simulink model "Model_14Bus_Microgrid_R2018"  (R2018b)
settings: Solver=ode23tb  StartTime=0.0  StopTime=0.35  MaxStep=1e-2  RelTol=1e-3
InitFcn:
  | Set_parameters_R2018
StopFcn:
  | Save_Data;
  | Graphics;
values from neighbouring files (symbols this model uses):
  Clink = Ceq*2    (= 0.217013888889)    [Set_parameters_R2017b.m]    (also in Set_parameters_R2018.m)
  dis1 = 0.15    [Set_parameters_R2017b.m]    (also in Set_parameters_R2018.m)
  dis10 = 6    [Set_parameters_R2017b.m]    (also in Set_parameters_R2018.m)
  dis11 = 3    [Set_parameters_R2017b.m]    (also in Set_parameters_R2018.m)
  dis12 = 6    [Set_parameters_R2017b.m]    (also in Set_parameters_R2018.m)
  dis13 = 3    [Set_parameters_R2017b.m]    (also in Set_parameters_R2018.m)
  dis14 = 2    [Set_parameters_R2017b.m]    (also in Set_parameters_R2018.m)
  dis2 = 0.2    [Set_parameters_R2017b.m]    (also in Set_parameters_R2018.m)
  dis3 = 0.15    [Set_parameters_R2017b.m]    (also in Set_parameters_R2018.m)
  dis4 = 0.4    [Set_parameters_R2017b.m]    (also in Set_parameters_R2018.m)
  dis5 = 0.4    [Set_parameters_R2017b.m]    (also in Set_parameters_R2018.m)
  dis6 = 0.4    [Set_parameters_R2017b.m]    (also in Set_parameters_R2018.m)
  dis7 = 0.1    [Set_parameters_R2017b.m]    (also in Set_parameters_R2018.m)
  dis8 = 2    [Set_parameters_R2017b.m]    (also in Set_parameters_R2018.m)
  dis9 = 6    [Set_parameters_R2017b.m]    (also in Set_parameters_R2018.m)
  Fc = 33 * Fnom    (= 1980)    [Set_parameters_R2017b.m]    (also in Set_parameters_R2018.m)
  Fnom = 60    [Main_DC_MG.m]    (also in Set_parameters_R2017b.m; Set_parameters_R2018.m)
  Increment_MPPT = 0.01    [Set_parameters_R2017b.m]    (also in Set_parameters_R2018.m)
  Ki_Ireg = 20    [Set_parameters_R2017b.m]    (also in Set_parameters_R2018.m)
  Ki_VDCreg = 400    [Set_parameters_R2017b.m]    (also in Set_parameters_R2018.m)
  Kp_Ireg = 0.3    [Set_parameters_R2017b.m]    (also in Set_parameters_R2018.m)
  Kp_VDCreg = 2    [Set_parameters_R2017b.m]    (also in Set_parameters_R2018.m)
  LimitL_Ireg = -1.5    [Set_parameters_R2017b.m]    (also in Set_parameters_R2018.m)
  LimitL_VDCreg = -1.5    [Set_parameters_R2017b.m]    (also in Set_parameters_R2018.m)
  Limits_MPPT = [ 583 357 ]    [Set_parameters_R2017b.m]    (also in Set_parameters_R2018.m)
  LimitU_Ireg = 1.5    [Set_parameters_R2017b.m]    (also in Set_parameters_R2018.m)
  LimitU_VDCreg = 1.5    [Set_parameters_R2017b.m]    (also in Set_parameters_R2018.m)
  P_Load_2 = S_Load_2* PF_Load_2    (= 36000)    [Set_parameters_R2017b.m]    (also in Set_parameters_R2018.m)
  P_Load_3 = S_Load_3* PF_Load_3    (= 25500)    [Set_parameters_R2017b.m]    (also in Set_parameters_R2018.m)
  Pnom = 1e6    (= 1000000)    [Set_parameters_R2017b.m]    (also in Set_parameters_R2018.m)
  Pnom_T1 = 1.5e6    (= 1500000)    [Set_parameters_R2017b.m]    (also in Set_parameters_R2018.m)
  Pnom_T2 = 1.5e6    (= 1500000)    [Set_parameters_R2017b.m]    (also in Set_parameters_R2018.m)
  Pnom_T3 = 4e6    (= 4000000)    [Set_parameters_R2017b.m]    (also in Set_parameters_R2018.m)
  Pnom_xfo = Pnom    (= 1000000)    [Set_parameters_R2017b.m]    (also in Set_parameters_R2018.m)
  Ql_Load_2 = S_Load_2 * sin(acos(PF_Load_2))    [Set_parameters_R2017b.m]    (also in Set_parameters_R2018.m)
  Ql_Load_3 = S_Load_3 * sin(acos(PF_Load_3))    [Set_parameters_R2017b.m]    (also in Set_parameters_R2018.m)
  R_Load_9 = (Vnom_prim * 1.35)^2 / P_Load_9    (= 1084.6153125)    [Set_parameters_R2017b.m]    (also in Set_parameters_R2018.m)
  R_Load_DC = Vnom_DC^2/ P_Load_DC    (= 45)    [Main_DC_MG.m]    (also in Set_parameters_R2017b.m; Set_parameters_R2018.m)
  Rl = 0.394    [Set_parameters_R2017b.m]    (also in Set_parameters_R2018.m)
  Rls = 0.198    [Set_parameters_R2017b.m]    (also in Set_parameters_R2018.m)
  Ts = Ts_Power    (= 5.05050505051e-06)    [Main_DC_MG.m]    (also in Set_parameters_R2017b.m; Set_parameters_R2018.m)
  Ts_Control = 10*Ts_Power    (= 5.05050505051e-05)    [Main_DC_MG.m]    (also in Set_parameters_R2017b.m; Set_parameters_R2018.m)
  Ts_Power = 1/(33*Fnom)/100    (= 5.05050505051e-06)    [Main_DC_MG.m]    (also in Set_parameters_R2017b.m; Set_parameters_R2018.m)
  V1_LL_T3 = 69e3    (= 69000)    [Set_parameters_R2017b.m]    (also in Set_parameters_R2018.m)
  Vf = 0    [Set_parameters_R2017b.m]    (also in Set_parameters_R2018.m)
  Vfd = 0    [Set_parameters_R2017b.m]    (also in Set_parameters_R2018.m)
  Vnom_DC = 300    [Main_DC_MG.m]    (also in Set_parameters_R2017b.m; Set_parameters_R2018.m)
  Vnom_dc = 480    [Set_parameters_R2017b.m]    (also in Set_parameters_R2018.m)
  Vnom_Diesel = 2.4e3    (= 2400)    [Set_parameters_R2017b.m]    (also in Set_parameters_R2018.m)
  Vnom_prim = 13.8e3    (= 13800)    [Set_parameters_R2017b.m]    (also in Set_parameters_R2018.m)
  Vnom_sec = 220    [Set_parameters_R2017b.m]    (also in Set_parameters_R2018.m)
  Vnom_ter_AC_DC = 150    [Set_parameters_R2017b.m]    (also in Set_parameters_R2018.m)
  Xl = 0.1168    [Set_parameters_R2017b.m]    (also in Set_parameters_R2018.m)
  Xls = 0.1089    [Set_parameters_R2017b.m]    (also in Set_parameters_R2018.m)
undefined symbols (not defined in the file or in its folder): D1, Delta, Hydride, Ion, Lithium, max_min, Metal, Nickel, RL, RLff, sigbuilder_block
libraries: powerlib x202, powerlib_meascontrol x152, simulink x14, powerlib_extras x14, electricdrivelib x4, re_lib x2
(part 3 of 10)

== system Model_14Bus_Microgrid_R2018/Bus_14 4 ==
  " r1_ L13" : Constant  Value=Rls
  Active powers losses A : Display
      settings: Format=bank
  Active powers losses B : Display
      settings: Format=bank
  Active powers losses c : Display
      settings: Format=bank
  "Delta Pabc " : Scope  NumInputPorts=4
  Math Function : Math  Operator=square  SaturateOnIntegerOverflow=on
  Math Function1 : Math  Operator=square  SaturateOnIntegerOverflow=on
  Math Function2 : Math  Operator=square  SaturateOnIntegerOverflow=on
  Mux : Mux  Inputs=3
  Product : Product
  Product1 : Product
  Product2 : Product
  RMS1 : powerlib_meascontrol/Measurements/RMS  TrueRMS=on  Freq=60  RMSInit=0  Ts=0
      settings: SourceProductName=Simscape Electrical
  RMS2 : powerlib_meascontrol/Measurements/RMS  TrueRMS=on  Freq=60  RMSInit=0  Ts=0
      settings: SourceProductName=Simscape Electrical
  RMS3 : powerlib_meascontrol/Measurements/RMS  TrueRMS=on  Freq=60  RMSInit=0  Ts=0
      settings: SourceProductName=Simscape Electrical
  W_to_kW : Gain  Gain=1e-3
  W_to_kW1 : Gain  Gain=1e-3
  W_to_kW2 : Gain  Gain=1e-3
  tag scope: Power_Losse_abc_L6=global
  wires:
  Math Function/1 -> Product/2
  [Ia_L6] -> RMS2/1
  Math Function1/1 -> Product1/2
  [Ib_L6] -> RMS1/1
  Math Function2/1 -> Product2/2
  " r1_ L13"/1 -> Product2/1, Product1/1, Product/1
  [Ic_L6] -> RMS3/1
  Product/1 -> W_to_kW/1
  Product2/1 -> W_to_kW2/1
  Product1/1 -> W_to_kW1/1
  RMS2/1 -> Math Function/1
  RMS1/1 -> Math Function1/1
  RMS3/1 -> Math Function2/1
  W_to_kW/1 -> Mux/1, "Delta Pabc "/1, Active powers losses A/1  "D_Pa_kW"
  W_to_kW1/1 -> Mux/2, "Delta Pabc "/2, Active powers losses B/1  "D_Pb_kW"
  W_to_kW2/1 -> Active powers losses c/1, Mux/3, "Delta Pabc "/3  "D_Pc_kW"
  Mux/1 -> [Power_Losse_abc_L6], "Delta Pabc "/4

== system Model_14Bus_Microgrid_R2018/Bus_14 5 ==
  " r1_ L13" : Constant  Value=Rls
  Active powers losses A : Display
      settings: Format=bank
  Active powers losses B : Display
      settings: Format=bank
  Active powers losses c : Display
      settings: Format=bank
  "Delta Pabc " : Scope  NumInputPorts=4
  Math Function : Math  Operator=square  SaturateOnIntegerOverflow=on
  Math Function1 : Math  Operator=square  SaturateOnIntegerOverflow=on
  Math Function2 : Math  Operator=square  SaturateOnIntegerOverflow=on
  Mux : Mux  Inputs=3
  Product : Product
  Product1 : Product
  Product2 : Product
  RMS1 : powerlib_meascontrol/Measurements/RMS  TrueRMS=on  Freq=60  RMSInit=0  Ts=0
      settings: SourceProductName=Simscape Electrical
  RMS2 : powerlib_meascontrol/Measurements/RMS  TrueRMS=on  Freq=60  RMSInit=0  Ts=0
      settings: SourceProductName=Simscape Electrical
  RMS3 : powerlib_meascontrol/Measurements/RMS  TrueRMS=on  Freq=60  RMSInit=0  Ts=0
      settings: SourceProductName=Simscape Electrical
  W_to_kW : Gain  Gain=1e-3
  W_to_kW1 : Gain  Gain=1e-3
  W_to_kW2 : Gain  Gain=1e-3
  tag scope: Power_Losse_abc_L5=global
  wires:
  Math Function/1 -> Product/2
  [Ia_L5] -> RMS2/1
  Math Function1/1 -> Product1/2
  [Ib_L5] -> RMS1/1
  Math Function2/1 -> Product2/2
  " r1_ L13"/1 -> Product2/1, Product1/1, Product/1
  [Ic_L5] -> RMS3/1
  Product/1 -> W_to_kW/1
  Product2/1 -> W_to_kW2/1
  Product1/1 -> W_to_kW1/1
  RMS2/1 -> Math Function/1
  RMS1/1 -> Math Function1/1
  RMS3/1 -> Math Function2/1
  W_to_kW/1 -> Mux/1, "Delta Pabc "/1, Active powers losses A/1  "D_Pa_kW"
  W_to_kW1/1 -> Mux/2, "Delta Pabc "/2, Active powers losses B/1  "D_Pb_kW"
  W_to_kW2/1 -> Active powers losses c/1, Mux/3, "Delta Pabc "/3  "D_Pc_kW"
  Mux/1 -> [Power_Losse_abc_L5], "Delta Pabc "/4

== system Model_14Bus_Microgrid_R2018/Bus_14 6 ==
  " r1_ L13" : Constant  Value=Rls
  Active powers losses A : Display
      settings: Format=bank
  Active powers losses B : Display
      settings: Format=bank
  Active powers losses c : Display
      settings: Format=bank
  "Delta Pabc " : Scope  NumInputPorts=4
  Math Function : Math  Operator=square  SaturateOnIntegerOverflow=on
  Math Function1 : Math  Operator=square  SaturateOnIntegerOverflow=on
  Math Function2 : Math  Operator=square  SaturateOnIntegerOverflow=on
  Mux : Mux  Inputs=3
  Product : Product
  Product1 : Product
  Product2 : Product
  RMS1 : powerlib_meascontrol/Measurements/RMS  TrueRMS=on  Freq=60  RMSInit=0  Ts=0
      settings: SourceProductName=Simscape Electrical
  RMS2 : powerlib_meascontrol/Measurements/RMS  TrueRMS=on  Freq=60  RMSInit=0  Ts=0
      settings: SourceProductName=Simscape Electrical
  RMS3 : powerlib_meascontrol/Measurements/RMS  TrueRMS=on  Freq=60  RMSInit=0  Ts=0
      settings: SourceProductName=Simscape Electrical
  W_to_kW : Gain  Gain=1e-3
  W_to_kW1 : Gain  Gain=1e-3
  W_to_kW2 : Gain  Gain=1e-3
  tag scope: Power_Losse_abc_L4=global
  wires:
  Math Function/1 -> Product/2
  [Ia_L4] -> RMS2/1
  Math Function1/1 -> Product1/2
  [Ib_L4] -> RMS1/1
  Math Function2/1 -> Product2/2
  " r1_ L13"/1 -> Product2/1, Product1/1, Product/1
  [Ic_L4] -> RMS3/1
  Product/1 -> W_to_kW/1
  Product2/1 -> W_to_kW2/1
  Product1/1 -> W_to_kW1/1
  RMS2/1 -> Math Function/1
  RMS1/1 -> Math Function1/1
  RMS3/1 -> Math Function2/1
  W_to_kW/1 -> Mux/1, "Delta Pabc "/1, Active powers losses A/1  "D_Pa_kW"
  W_to_kW1/1 -> Mux/2, "Delta Pabc "/2, Active powers losses B/1  "D_Pb_kW"
  W_to_kW2/1 -> Active powers losses c/1, Mux/3, "Delta Pabc "/3  "D_Pc_kW"
  Mux/1 -> [Power_Losse_abc_L4], "Delta Pabc "/4

== system Model_14Bus_Microgrid_R2018/Bus_14 7 ==
  " r1_ L13" : Constant  Value=Rls
  Active powers losses A : Display
      settings: Format=bank
  Active powers losses B : Display
      settings: Format=bank
  Active powers losses c : Display
      settings: Format=bank
  "Delta Pabc " : Scope  NumInputPorts=4
  Math Function : Math  Operator=square  SaturateOnIntegerOverflow=on
  Math Function1 : Math  Operator=square  SaturateOnIntegerOverflow=on
  Math Function2 : Math  Operator=square  SaturateOnIntegerOverflow=on
  Mux : Mux  Inputs=3
  Product : Product
  Product1 : Product
  Product2 : Product
  RMS1 : powerlib_meascontrol/Measurements/RMS  TrueRMS=on  Freq=60  RMSInit=0  Ts=0
      settings: SourceProductName=Simscape Electrical
  RMS2 : powerlib_meascontrol/Measurements/RMS  TrueRMS=on  Freq=60  RMSInit=0  Ts=0
      settings: SourceProductName=Simscape Electrical
  RMS3 : powerlib_meascontrol/Measurements/RMS  TrueRMS=on  Freq=60  RMSInit=0  Ts=0
      settings: SourceProductName=Simscape Electrical
  W_to_kW : Gain  Gain=1e-3
  W_to_kW1 : Gain  Gain=1e-3
  W_to_kW2 : Gain  Gain=1e-3
  tag scope: Power_Losse_abc_L3=global
  wires:
  Math Function/1 -> Product/2
  [Ia_L3] -> RMS2/1
  Math Function1/1 -> Product1/2
  [Ib_L3] -> RMS1/1
  Math Function2/1 -> Product2/2
  " r1_ L13"/1 -> Product2/1, Product1/1, Product/1
  [Ic_L3] -> RMS3/1
  Product/1 -> W_to_kW/1
  Product2/1 -> W_to_kW2/1
  Product1/1 -> W_to_kW1/1
  RMS2/1 -> Math Function/1
  RMS1/1 -> Math Function1/1
  RMS3/1 -> Math Function2/1
  W_to_kW/1 -> Mux/1, "Delta Pabc "/1, Active powers losses A/1  "D_Pa_kW"
  W_to_kW1/1 -> Mux/2, "Delta Pabc "/2, Active powers losses B/1  "D_Pb_kW"
  W_to_kW2/1 -> Active powers losses c/1, Mux/3, "Delta Pabc "/3  "D_Pc_kW"
  Mux/1 -> [Power_Losse_abc_L3], "Delta Pabc "/4

== system Model_14Bus_Microgrid_R2018/Bus_14 8 ==
  " r1_ L13" : Constant  Value=Rls
  Active powers losses A : Display
      settings: Format=bank
  Active powers losses B : Display
      settings: Format=bank
  Active powers losses c : Display
      settings: Format=bank
  "Delta Pabc " : Scope  NumInputPorts=4
  Math Function : Math  Operator=square  SaturateOnIntegerOverflow=on
  Math Function1 : Math  Operator=square  SaturateOnIntegerOverflow=on
  Math Function2 : Math  Operator=square  SaturateOnIntegerOverflow=on
  Mux : Mux  Inputs=3
  Product : Product
  Product1 : Product
  Product2 : Product
  RMS1 : powerlib_meascontrol/Measurements/RMS  TrueRMS=on  Freq=60  RMSInit=0  Ts=0
      settings: SourceProductName=Simscape Electrical
  RMS2 : powerlib_meascontrol/Measurements/RMS  TrueRMS=on  Freq=60  RMSInit=0  Ts=0
      settings: SourceProductName=Simscape Electrical
  RMS3 : powerlib_meascontrol/Measurements/RMS  TrueRMS=on  Freq=60  RMSInit=0  Ts=0
      settings: SourceProductName=Simscape Electrical
  W_to_kW : Gain  Gain=1e-3
  W_to_kW1 : Gain  Gain=1e-3
  W_to_kW2 : Gain  Gain=1e-3
  tag scope: Power_Losse_abc_L7=global
  wires:
  Math Function/1 -> Product/2
  [Ia_L7] -> RMS2/1
  Math Function1/1 -> Product1/2
  [Ib_L7] -> RMS1/1
  Math Function2/1 -> Product2/2
  " r1_ L13"/1 -> Product2/1, Product1/1, Product/1
  [Ic_L7] -> RMS3/1
  Product/1 -> W_to_kW/1
  Product2/1 -> W_to_kW2/1
  Product1/1 -> W_to_kW1/1
  RMS2/1 -> Math Function/1
  RMS1/1 -> Math Function1/1
  RMS3/1 -> Math Function2/1
  W_to_kW/1 -> Mux/1, "Delta Pabc "/1, Active powers losses A/1  "D_Pa_kW"
  W_to_kW1/1 -> Mux/2, "Delta Pabc "/2, Active powers losses B/1  "D_Pb_kW"
  W_to_kW2/1 -> Active powers losses c/1, Mux/3, "Delta Pabc "/3  "D_Pc_kW"
  Mux/1 -> [Power_Losse_abc_L7], "Delta Pabc "/4

== system Model_14Bus_Microgrid_R2018/Bus_14 9 ==
  " r1_ L13" : Constant  Value=Rl
  Active powers losses A : Display
      settings: Format=bank
  Active powers losses B : Display
      settings: Format=bank
  Active powers losses c : Display
      settings: Format=bank
  "Delta Pabc " : Scope  NumInputPorts=4
  Math Function : Math  Operator=square  SaturateOnIntegerOverflow=on
  Math Function1 : Math  Operator=square  SaturateOnIntegerOverflow=on
  Math Function2 : Math  Operator=square  SaturateOnIntegerOverflow=on
  Mux : Mux  Inputs=3
  Product : Product
  Product1 : Product
  Product2 : Product
  RMS1 : powerlib_meascontrol/Measurements/RMS  TrueRMS=on  Freq=60  RMSInit=0  Ts=0
      settings: SourceProductName=Simscape Electrical
  RMS2 : powerlib_meascontrol/Measurements/RMS  TrueRMS=on  Freq=60  RMSInit=0  Ts=0
      settings: SourceProductName=Simscape Electrical
  RMS3 : powerlib_meascontrol/Measurements/RMS  TrueRMS=on  Freq=60  RMSInit=0  Ts=0
      settings: SourceProductName=Simscape Electrical
  W_to_kW : Gain  Gain=1e-3
  W_to_kW1 : Gain  Gain=1e-3
  W_to_kW2 : Gain  Gain=1e-3
  tag scope: Power_Losse_abc_L8=global
  wires:
  Math Function/1 -> Product/2
  [Ia_L8] -> RMS2/1
  Math Function1/1 -> Product1/2
  [Ib_L8] -> RMS1/1
  Math Function2/1 -> Product2/2
  " r1_ L13"/1 -> Product2/1, Product1/1, Product/1
  [Ic_L8] -> RMS3/1
  Product/1 -> W_to_kW/1
  Product2/1 -> W_to_kW2/1
  Product1/1 -> W_to_kW1/1
  RMS2/1 -> Math Function/1
  RMS1/1 -> Math Function1/1
  RMS3/1 -> Math Function2/1
  W_to_kW/1 -> Mux/1, "Delta Pabc "/1, Active powers losses A/1  "D_Pa_kW"
  W_to_kW1/1 -> Mux/2, "Delta Pabc "/2, Active powers losses B/1  "D_Pb_kW"
  W_to_kW2/1 -> Active powers losses c/1, Mux/3, "Delta Pabc "/3  "D_Pc_kW"
  Mux/1 -> [Power_Losse_abc_L8], "Delta Pabc "/4

== system Model_14Bus_Microgrid_R2018/Bus_2 ==
  note: C
  note: B
  note: A
  note: A
  note: B
  note: Linea - Neutro
  note: C
  note: A
  note: B
  note: C
  Conv pu1 : Gain  Gain=sqrt (3) /Vnom_sec  SaturateOnIntegerOverflow=on  OutDataTypeStr=Inherit: Same as input  ParamDataTypeStr=Inherit: Same as input
  Conv pu2 : Gain  Gain=sqrt (3) /Vnom_sec  SaturateOnIntegerOverflow=on  OutDataTypeStr=Inherit: Same as input  ParamDataTypeStr=Inherit: Same as input
  Measurement1 : Scope  NumInputPorts=4
  PLL : Subsystem
  PLL (3ph) : powerlib_meascontrol/PLL/PLL (3ph)  Fmin=45  Par_Init=[0, 60]  ParK=[180, 3200, 1]  TcD=1e-4  MaxRateChangeFreq=12  FilterCutOffFreq=25  Ts=0  AGC=on
      settings: SourceProductName=Simscape Electrical
  Power Factor Block1 : Subsystem  mask(Power Factor Block){Freq=Fnom, Vinit=[0, 0], Iinit=[0, 0], Ts=0}
      mask prompts: Freq "Fundamental frequency (Hz):"; Vinit "Voltage initial input [ Mag, Phase (degrees) ]:"; Iinit "Current initial input [ Mag, Phase (degrees) ]:"; Ts "Sample time:"
      mask help:
      | Power Factor Block developed by Dr Rodney Tan
      | Version 1.01 (Aug 2016)
      |
      | Compute power factor and phase angle of AC circuit voltage-current pair at fundamental frequency.
      |
      | The computation is based on Power block and Complex number function block.
      |
      | For the first cycle of simulation, the outputs are held constant to the powers computed for the Voltage initial input and Current initial input parameters.
      mask Help:
      | <b>Fundamental Frequency (Hz)</b>
      | Specify the measurement fundamental frequency, in hertz, of the input signal.
      | 
      | <b>Voltage initial input [ Mag, Phase (degrees) ]</b>
      | Specify the voltage initial magnitude and phase to set a constant output for the first cycle of simulation.
      | 
      | <b>Current initial input [ Mag, Phase (degrees) ]</b>
      | Specify the current initial magnitude and phase to set a constant output for the first cycle of simulation.
      | 
      | <b>Sample Time</b>
      | Specify the sample time of the block, in seconds. Set to 0 to implement a continuous block.
      mask TypeOptions Freq: Power/Freq
      mask TypeOptions Vinit: Power/Vinit
      mask TypeOptions Iinit: Power/Iinit
      mask TypeOptions Ts: Power/Ts
  Power Factor1 : Display
  Scope : Scope
  Scope2 : Scope
  THD : powerlib_meascontrol/Measurements/THD  Freq=60  Ts=Ts_Power
      settings: SourceProductName=Simscape Electrical
  THD (% and signal) : Scope  NumInputPorts=2
  THD (%) : Display
      settings: Format=bank
  Terminator : Terminator
  Vabc pu1 : Scope
  frecuency (Hz) : Display
  to % : Gain  Gain=100  SampleTime=Ts_Power
  ángulo de V (%)1 : Display
      settings: Format=bank
  tag scope: PFabc_Bus2=global, THDv_abc_Bus2=global, delta_abc_Bus2=global
  wires:
  [IabcLL_Bus_2] -> Power Factor Block1/2(Iabc)
  THD/1 -> to %/1
  Power Factor Block1/3(Vabc y Vabc (rms)) -> Conv pu1/1, Measurement1/3
  Power Factor Block1/4(Iabc y Iabc (rms)) -> Measurement1/4
  Conv pu1/1 -> Vabc pu1/1
  Power Factor Block1/2(Qabc) -> Measurement1/2
  Power Factor Block1/1(Pabc) -> Measurement1/1
  Power Factor Block1/5("PFabc ") -> [PFabc_Bus2], Power Factor1/1
  to %/1 -> [THDv_abc_Bus2], THD (%)/1, THD (% and signal)/2  "THD (%)"
  Conv pu2/1 -> PLL/1(Vabc_LN_pu)
  PLL/1(delta_abc) -> [delta_abc_Bus2], Scope/1, ángulo de V (%)1/1
  PLL (3ph)/2 -> Terminator/1
  [VabcLL_Bus_2] -> PLL (3ph)/1, Conv pu2/1, THD/1, THD (% and signal)/1, Power Factor Block1/1(Vabc)  "Vabc"
  PLL (3ph)/1 -> Scope2/1, frecuency (Hz)/1

== system Model_14Bus_Microgrid_R2018/Bus_3 ==
  note: C
  note: B
  note: A
  note: C
  note: Linea - Neutro
  note: B
  note: A
  note: A
  note: B
  note: C
  Conv pu1 : Gain  Gain=sqrt (3) /Vnom_sec  SaturateOnIntegerOverflow=on  OutDataTypeStr=Inherit: Same as input  ParamDataTypeStr=Inherit: Same as input
  Conv pu2 : Gain  Gain=sqrt (3) /Vnom_sec  SaturateOnIntegerOverflow=on  OutDataTypeStr=Inherit: Same as input  ParamDataTypeStr=Inherit: Same as input
  Measurement1 : Scope  NumInputPorts=4
  PLL : Subsystem
  Power Factor Block1 : Subsystem  mask(Power Factor Block){Freq=Fnom, Vinit=[0, 0], Iinit=[0, 0], Ts=0}
      mask prompts: Freq "Fundamental frequency (Hz):"; Vinit "Voltage initial input [ Mag, Phase (degrees) ]:"; Iinit "Current initial input [ Mag, Phase (degrees) ]:"; Ts "Sample time:"
      mask help:
      | Power Factor Block developed by Dr Rodney Tan
      | Version 1.01 (Aug 2016)
      |
      | Compute power factor and phase angle of AC circuit voltage-current pair at fundamental frequency.
      |
      | The computation is based on Power block and Complex number function block.
      |
      | For the first cycle of simulation, the outputs are held constant to the powers computed for the Voltage initial input and Current initial input parameters.
      mask Help:
      | <b>Fundamental Frequency (Hz)</b>
      | Specify the measurement fundamental frequency, in hertz, of the input signal.
      | 
      | <b>Voltage initial input [ Mag, Phase (degrees) ]</b>
      | Specify the voltage initial magnitude and phase to set a constant output for the first cycle of simulation.
      | 
      | <b>Current initial input [ Mag, Phase (degrees) ]</b>
      | Specify the current initial magnitude and phase to set a constant output for the first cycle of simulation.
      | 
      | <b>Sample Time</b>
      | Specify the sample time of the block, in seconds. Set to 0 to implement a continuous block.
      mask TypeOptions Freq: Power/Freq
      mask TypeOptions Vinit: Power/Vinit
      mask TypeOptions Iinit: Power/Iinit
      mask TypeOptions Ts: Power/Ts
  Power Factor1 : Display
  Scope : Scope
  THD : powerlib_meascontrol/Measurements/THD  Freq=60  Ts=Ts_Power
      settings: SourceProductName=Simscape Electrical
  THD (% and signal) : Scope  NumInputPorts=2
  THD (%) : Display
      settings: Format=bank
  Vabc pu1 : Scope
  to % : Gain  Gain=100  SampleTime=Ts_Power
  ángulo de V (%)1 : Display
      settings: Format=bank
  tag scope: PFabc_Bus3=global, THDv_abc_Bus3=global, delta_abc_Bus3=global
  wires:
  [IabcLL_Bus_3] -> Power Factor Block1/2(Iabc)
  THD/1 -> to %/1
  Power Factor Block1/4(Iabc y Iabc (rms)) -> Measurement1/4
  Power Factor Block1/1(Pabc) -> Measurement1/1
  Conv pu1/1 -> Vabc pu1/1
  Power Factor Block1/2(Qabc) -> Measurement1/2
  Power Factor Block1/3(Vabc y Vabc (rms)) -> Conv pu1/1, Measurement1/3
  Power Factor Block1/5("PFabc ") -> [PFabc_Bus3], Power Factor1/1
  to %/1 -> [THDv_abc_Bus3], THD (%)/1, THD (% and signal)/2  "THD (%)"
  Conv pu2/1 -> PLL/1(Vabc_LN_pu)
  PLL/1(delta_abc) -> [delta_abc_Bus3], Scope/1, ángulo de V (%)1/1
  [VabcLL_Bus_3] -> Conv pu2/1, THD/1, THD (% and signal)/1, Power Factor Block1/1(Vabc)  "Signal Vabc"

== system Model_14Bus_Microgrid_R2018/Bus_4 ==
  note: C
  note: B
  note: A
  note: C
  note: Linea - Neutro
  note: B
  note: A
  note: A
  note: B
  note: C
  Conv pu1 : Gain  Gain=sqrt (3) /Vnom_sec  SaturateOnIntegerOverflow=on  OutDataTypeStr=Inherit: Same as input  ParamDataTypeStr=Inherit: Same as input
  Conv pu2 : Gain  Gain=sqrt (3) /Vnom_sec  SaturateOnIntegerOverflow=on  OutDataTypeStr=Inherit: Same as input  ParamDataTypeStr=Inherit: Same as input
  Measurement1 : Scope  NumInputPorts=4
  PLL : Subsystem
  Power Factor Block1 : Subsystem  mask(Power Factor Block){Freq=Fnom, Vinit=[0, 0], Iinit=[0, 0], Ts=0}
      mask prompts: Freq "Fundamental frequency (Hz):"; Vinit "Voltage initial input [ Mag, Phase (degrees) ]:"; Iinit "Current initial input [ Mag, Phase (degrees) ]:"; Ts "Sample time:"
      mask help:
      | Power Factor Block developed by Dr Rodney Tan
      | Version 1.01 (Aug 2016)
      |
      | Compute power factor and phase angle of AC circuit voltage-current pair at fundamental frequency.
      |
      | The computation is based on Power block and Complex number function block.
      |
      | For the first cycle of simulation, the outputs are held constant to the powers computed for the Voltage initial input and Current initial input parameters.
      mask Help:
      | <b>Fundamental Frequency (Hz)</b>
      | Specify the measurement fundamental frequency, in hertz, of the input signal.
      | 
      | <b>Voltage initial input [ Mag, Phase (degrees) ]</b>
      | Specify the voltage initial magnitude and phase to set a constant output for the first cycle of simulation.
      | 
      | <b>Current initial input [ Mag, Phase (degrees) ]</b>
      | Specify the current initial magnitude and phase to set a constant output for the first cycle of simulation.
      | 
      | <b>Sample Time</b>
      | Specify the sample time of the block, in seconds. Set to 0 to implement a continuous block.
      mask TypeOptions Freq: Power/Freq
      mask TypeOptions Vinit: Power/Vinit
      mask TypeOptions Iinit: Power/Iinit
      mask TypeOptions Ts: Power/Ts
  Power Factor1 : Display
  Scope : Scope
  THD : powerlib_meascontrol/Measurements/THD  Freq=60  Ts=Ts_Power
      settings: SourceProductName=Simscape Electrical
  THD (% and signal) : Scope  NumInputPorts=2
  THD (%) : Display
      settings: Format=bank
  Vabc pu1 : Scope
  to % : Gain  Gain=100  SampleTime=Ts_Power
  ángulo de V (%)1 : Display
      settings: Format=bank
  tag scope: PFabc_Bus4=global, THDv_abc_Bus4=global, delta_abc_Bus4=global
  wires:
  [IabcLL_Bus_4] -> Power Factor Block1/2(Iabc)
  THD/1 -> to %/1
  Power Factor Block1/4(Iabc y Iabc (rms)) -> Measurement1/4
  Power Factor Block1/1(Pabc) -> Measurement1/1
  Conv pu1/1 -> Vabc pu1/1
  Power Factor Block1/2(Qabc) -> Measurement1/2
  Power Factor Block1/3(Vabc y Vabc (rms)) -> Conv pu1/1, Measurement1/3
  Power Factor Block1/5("PFabc ") -> [PFabc_Bus4], Power Factor1/1
  to %/1 -> [THDv_abc_Bus4], THD (%)/1, THD (% and signal)/2  "THD (%)"
  Conv pu2/1 -> PLL/1(Vabc_LN_pu)
  PLL/1(delta_abc) -> [delta_abc_Bus4], Scope/1, ángulo de V (%)1/1
  [VabcLL_Bus_4] -> Power Factor Block1/1(Vabc), Conv pu2/1, THD/1, THD (% and signal)/1  "Signal Vabc"

== system Model_14Bus_Microgrid_R2018/Bus_5 ==
  note: C
  note: B
  note: A
  note: C
  note: Linea - Neutro
  note: B
  note: A
  note: A
  note: B
  note: C
  Conv pu1 : Gain  Gain=sqrt (3) /Vnom_sec  SaturateOnIntegerOverflow=on  OutDataTypeStr=Inherit: Same as input  ParamDataTypeStr=Inherit: Same as input
  Conv pu2 : Gain  Gain=sqrt (3) /Vnom_sec  SaturateOnIntegerOverflow=on  OutDataTypeStr=Inherit: Same as input  ParamDataTypeStr=Inherit: Same as input
  Measurement1 : Scope  NumInputPorts=4
  PLL : Subsystem
  Power Factor Block1 : Subsystem  mask(Power Factor Block){Freq=Fnom, Vinit=[0, 0], Iinit=[0, 0], Ts=0}
      mask prompts: Freq "Fundamental frequency (Hz):"; Vinit "Voltage initial input [ Mag, Phase (degrees) ]:"; Iinit "Current initial input [ Mag, Phase (degrees) ]:"; Ts "Sample time:"
      mask help:
      | Power Factor Block developed by Dr Rodney Tan
      | Version 1.01 (Aug 2016)
      |
      | Compute power factor and phase angle of AC circuit voltage-current pair at fundamental frequency.
      |
      | The computation is based on Power block and Complex number function block.
      |
      | For the first cycle of simulation, the outputs are held constant to the powers computed for the Voltage initial input and Current initial input parameters.
      mask Help:
      | <b>Fundamental Frequency (Hz)</b>
      | Specify the measurement fundamental frequency, in hertz, of the input signal.
      | 
      | <b>Voltage initial input [ Mag, Phase (degrees) ]</b>
      | Specify the voltage initial magnitude and phase to set a constant output for the first cycle of simulation.
      | 
      | <b>Current initial input [ Mag, Phase (degrees) ]</b>
      | Specify the current initial magnitude and phase to set a constant output for the first cycle of simulation.
      | 
      | <b>Sample Time</b>
      | Specify the sample time of the block, in seconds. Set to 0 to implement a continuous block.
      mask TypeOptions Freq: Power/Freq
      mask TypeOptions Vinit: Power/Vinit
      mask TypeOptions Iinit: Power/Iinit
      mask TypeOptions Ts: Power/Ts
  Power Factor1 : Display
  Scope : Scope
  THD : powerlib_meascontrol/Measurements/THD  Freq=60  Ts=Ts_Power
      settings: SourceProductName=Simscape Electrical
  THD (% and signal) : Scope  NumInputPorts=2
  THD (%) : Display
      settings: Format=bank
  Vabc pu1 : Scope
  to % : Gain  Gain=100  SampleTime=Ts_Power
  ángulo de V (%)1 : Display
      settings: Format=bank
  tag scope: PFabc_Bus5=global, THDv_abc_Bus5=global, delta_abc_Bus5=global
  wires:
  [IabcLL_Bus_5] -> Power Factor Block1/2(Iabc)
  THD/1 -> to %/1
  Power Factor Block1/4(Iabc y Iabc (rms)) -> Measurement1/4
  Power Factor Block1/1(Pabc) -> Measurement1/1
  Conv pu1/1 -> Vabc pu1/1
  Power Factor Block1/2(Qabc) -> Measurement1/2
  Power Factor Block1/3(Vabc y Vabc (rms)) -> Conv pu1/1, Measurement1/3
  Power Factor Block1/5("PFabc ") -> [PFabc_Bus5], Power Factor1/1
  to %/1 -> [THDv_abc_Bus5], THD (%)/1, THD (% and signal)/2  "THD (%)"
  Conv pu2/1 -> PLL/1(Vabc_LN_pu)
  PLL/1(delta_abc) -> [delta_abc_Bus5], Scope/1, ángulo de V (%)1/1
  [VabcLL_Bus_5] -> Power Factor Block1/1(Vabc), Conv pu2/1, THD/1, THD (% and signal)/1  "Signal Vabc"

== system Model_14Bus_Microgrid_R2018/Bus_6  ==
  note: C
  note: B
  note: A
  note: C
  note: Linea - Neutro
  note: B
  note: A
  note: A
  note: B
  Conv pu1 : Gain  Gain=sqrt (3) /Vnom_prim  SaturateOnIntegerOverflow=on  OutDataTypeStr=Inherit: Same as input  ParamDataTypeStr=Inherit: Same as input
  Conv pu2 : Gain  Gain=sqrt (3) /Vnom_prim  SaturateOnIntegerOverflow=on  OutDataTypeStr=Inherit: Same as input  ParamDataTypeStr=Inherit: Same as input
  Measurement1 : Scope  NumInputPorts=4
  PLL : Subsystem
  PLL (3ph) : powerlib_meascontrol/PLL/PLL (3ph)  Fmin=45  Par_Init=[0, 60]  ParK=[180, 3200, 1]  TcD=1e-4  MaxRateChangeFreq=12  FilterCutOffFreq=25  Ts=0  AGC=on
      settings: SourceProductName=Simscape Electrical
  Power Factor Block1 : Subsystem  mask(Power Factor Block){Freq=Fnom, Vinit=[0, 0], Iinit=[0, 0], Ts=0}
      mask prompts: Freq "Fundamental frequency (Hz):"; Vinit "Voltage initial input [ Mag, Phase (degrees) ]:"; Iinit "Current initial input [ Mag, Phase (degrees) ]:"; Ts "Sample time:"
      mask help:
      | Power Factor Block developed by Dr Rodney Tan
      | Version 1.01 (Aug 2016)
      |
      | Compute power factor and phase angle of AC circuit voltage-current pair at fundamental frequency.
      |
      | The computation is based on Power block and Complex number function block.
      |
      | For the first cycle of simulation, the outputs are held constant to the powers computed for the Voltage initial input and Current initial input parameters.
      mask Help:
      | <b>Fundamental Frequency (Hz)</b>
      | Specify the measurement fundamental frequency, in hertz, of the input signal.
      | 
      | <b>Voltage initial input [ Mag, Phase (degrees) ]</b>
      | Specify the voltage initial magnitude and phase to set a constant output for the first cycle of simulation.
      | 
      | <b>Current initial input [ Mag, Phase (degrees) ]</b>
      | Specify the current initial magnitude and phase to set a constant output for the first cycle of simulation.
      | 
      | <b>Sample Time</b>
      | Specify the sample time of the block, in seconds. Set to 0 to implement a continuous block.
      mask TypeOptions Freq: Power/Freq
      mask TypeOptions Vinit: Power/Vinit
      mask TypeOptions Iinit: Power/Iinit
      mask TypeOptions Ts: Power/Ts
  Power Factor1 : Display
  Scope : Scope
  Scope2 : Scope
  THD : powerlib_meascontrol/Measurements/THD  Freq=60  Ts=Ts_Power
      settings: SourceProductName=Simscape Electrical
  THD (% and signal) : Scope  NumInputPorts=2
  THD (%) : Display
      settings: Format=bank
  Terminator : Terminator
  Vabc pu1 : Scope
  frecuency (Hz) : Display
  to % : Gain  Gain=100  SampleTime=Ts_Power
  ángulo de V (%)1 : Display
      settings: Format=bank
  tag scope: PFabc_Bus6=global, THDv_abc_Bus6=global, delta_abc_Bus6=global
  wires:
  [IabcLL_Bus_6] -> Power Factor Block1/2(Iabc)
  THD/1 -> to %/1
  Power Factor Block1/4(Iabc y Iabc (rms)) -> Measurement1/4
  Power Factor Block1/1(Pabc) -> Measurement1/1
  Conv pu1/1 -> Vabc pu1/1
  Power Factor Block1/2(Qabc) -> Measurement1/2
  Power Factor Block1/3(Vabc y Vabc (rms)) -> Conv pu1/1, Measurement1/3
  Power Factor Block1/5("PFabc ") -> [PFabc_Bus6], Power Factor1/1
  to %/1 -> [THDv_abc_Bus6], THD (%)/1, THD (% and signal)/2  "THD (%)"
  PLL/1(delta_abc) -> [delta_abc_Bus6], Scope/1, ángulo de V (%)1/1
  Conv pu2/1 -> PLL/1(Vabc_LN_pu)
  PLL (3ph)/2 -> Terminator/1
  [VabcLL_Bus_6] -> Power Factor Block1/1(Vabc), Conv pu2/1, PLL (3ph)/1, THD/1, THD (% and signal)/1  "Vabc"
  PLL (3ph)/1 -> Scope2/1, frecuency (Hz)/1

== system Model_14Bus_Microgrid_R2018/Bus_7 ==
  note: C
  note: B
  note: A
  note: C
  note: Linea - Neutro
  note: B
  note: A
  note: A
  note: B
  Conv pu1 : Gain  Gain=sqrt (3) /Vnom_prim  SaturateOnIntegerOverflow=on  OutDataTypeStr=Inherit: Same as input  ParamDataTypeStr=Inherit: Same as input
  Conv pu2 : Gain  Gain=sqrt (3) /Vnom_prim  SaturateOnIntegerOverflow=on  OutDataTypeStr=Inherit: Same as input  ParamDataTypeStr=Inherit: Same as input
  Measurement1 : Scope  NumInputPorts=4
  PLL : Subsystem
  PLL (3ph) : powerlib_meascontrol/PLL/PLL (3ph)  Fmin=45  Par_Init=[0, 60]  ParK=[180, 3200, 1]  TcD=1e-4  MaxRateChangeFreq=12  FilterCutOffFreq=25  Ts=0  AGC=on
      settings: SourceProductName=Simscape Electrical
  Power Factor Block1 : Subsystem  mask(Power Factor Block){Freq=Fnom, Vinit=[0, 0], Iinit=[0, 0], Ts=0}
      mask prompts: Freq "Fundamental frequency (Hz):"; Vinit "Voltage initial input [ Mag, Phase (degrees) ]:"; Iinit "Current initial input [ Mag, Phase (degrees) ]:"; Ts "Sample time:"
      mask help:
      | Power Factor Block developed by Dr Rodney Tan
      | Version 1.01 (Aug 2016)
      |
      | Compute power factor and phase angle of AC circuit voltage-current pair at fundamental frequency.
      |
      | The computation is based on Power block and Complex number function block.
      |
      | For the first cycle of simulation, the outputs are held constant to the powers computed for the Voltage initial input and Current initial input parameters.
      mask Help:
      | <b>Fundamental Frequency (Hz)</b>
      | Specify the measurement fundamental frequency, in hertz, of the input signal.
      | 
      | <b>Voltage initial input [ Mag, Phase (degrees) ]</b>
      | Specify the voltage initial magnitude and phase to set a constant output for the first cycle of simulation.
      | 
      | <b>Current initial input [ Mag, Phase (degrees) ]</b>
      | Specify the current initial magnitude and phase to set a constant output for the first cycle of simulation.
      | 
      | <b>Sample Time</b>
      | Specify the sample time of the block, in seconds. Set to 0 to implement a continuous block.
      mask TypeOptions Freq: Power/Freq
      mask TypeOptions Vinit: Power/Vinit
      mask TypeOptions Iinit: Power/Iinit
      mask TypeOptions Ts: Power/Ts
  Power Factor1 : Display
  Scope : Scope
  Scope2 : Scope
  THD : powerlib_meascontrol/Measurements/THD  Freq=60  Ts=Ts_Power
      settings: SourceProductName=Simscape Electrical
  THD (% and signal) : Scope  NumInputPorts=2
  THD (%) : Display
      settings: Format=bank
  Terminator : Terminator
  Vabc pu1 : Scope
  frecuency (Hz) : Display
  to % : Gain  Gain=100  SampleTime=Ts_Power
  ángulo de V (%)1 : Display
      settings: Format=bank
  tag scope: PFabc_Bus7=global, THDv_abc_Bus7=global, delta_abc_Bus7=global
  wires:
  [IabcLL_Bus_7] -> Power Factor Block1/2(Iabc)
  THD/1 -> to %/1
  Power Factor Block1/4(Iabc y Iabc (rms)) -> Measurement1/4
  Power Factor Block1/1(Pabc) -> Measurement1/1
  Conv pu1/1 -> Vabc pu1/1
  Power Factor Block1/2(Qabc) -> Measurement1/2
  Power Factor Block1/3(Vabc y Vabc (rms)) -> Conv pu1/1, Measurement1/3
  to %/1 -> [THDv_abc_Bus7], THD (%)/1, THD (% and signal)/2  "THD (%)"
  Power Factor Block1/5("PFabc ") -> [PFabc_Bus7], Power Factor1/1
  PLL/1(delta_abc) -> [delta_abc_Bus7], Scope/1, ángulo de V (%)1/1
  Conv pu2/1 -> PLL/1(Vabc_LN_pu)
  [VabcLL_Bus_7] -> PLL (3ph)/1, Conv pu2/1, THD/1, THD (% and signal)/1, Power Factor Block1/1(Vabc)  "Vabc"
  PLL (3ph)/2 -> Terminator/1
  PLL (3ph)/1 -> Scope2/1, frecuency (Hz)/1

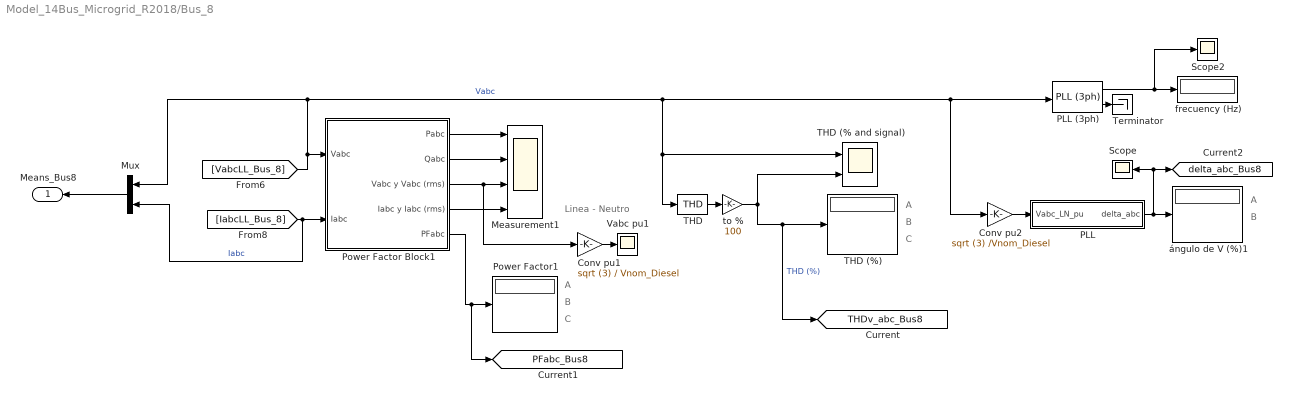
== system Model_14Bus_Microgrid_R2018/Bus_8       ==
  note: C
  note: B
  note: A
  note: C
  note: Linea - Neutro
  note: B
  note: A
  note: A
  note: B
  Conv pu1 : Gain  Gain=sqrt (3) / Vnom_Diesel  SaturateOnIntegerOverflow=on  OutDataTypeStr=Inherit: Same as input  ParamDataTypeStr=Inherit: Same as input
  Conv pu2 : Gain  Gain=sqrt (3) /Vnom_Diesel  SaturateOnIntegerOverflow=on  OutDataTypeStr=Inherit: Same as input  ParamDataTypeStr=Inherit: Same as input
  Measurement1 : Scope  NumInputPorts=4
  Mux : Mux  Inputs=2
  PLL : Subsystem
  PLL (3ph) : powerlib_meascontrol/PLL/PLL (3ph)  Fmin=45  Par_Init=[0, 60]  ParK=[180, 3200, 1]  TcD=1e-4  MaxRateChangeFreq=12  FilterCutOffFreq=25  Ts=0  AGC=on
      settings: SourceProductName=Simscape Electrical
  Power Factor Block1 : Subsystem  mask(Power Factor Block){Freq=Fnom, Vinit=[0, 0], Iinit=[0, 0], Ts=0}
      mask prompts: Freq "Fundamental frequency (Hz):"; Vinit "Voltage initial input [ Mag, Phase (degrees) ]:"; Iinit "Current initial input [ Mag, Phase (degrees) ]:"; Ts "Sample time:"
      mask help:
      | Power Factor Block developed by Dr Rodney Tan
      | Version 1.01 (Aug 2016)
      |
      | Compute power factor and phase angle of AC circuit voltage-current pair at fundamental frequency.
      |
      | The computation is based on Power block and Complex number function block.
      |
      | For the first cycle of simulation, the outputs are held constant to the powers computed for the Voltage initial input and Current initial input parameters.
      mask Help:
      | <b>Fundamental Frequency (Hz)</b>
      | Specify the measurement fundamental frequency, in hertz, of the input signal.
      | 
      | <b>Voltage initial input [ Mag, Phase (degrees) ]</b>
      | Specify the voltage initial magnitude and phase to set a constant output for the first cycle of simulation.
      | 
      | <b>Current initial input [ Mag, Phase (degrees) ]</b>
      | Specify the current initial magnitude and phase to set a constant output for the first cycle of simulation.
      | 
      | <b>Sample Time</b>
      | Specify the sample time of the block, in seconds. Set to 0 to implement a continuous block.
      mask TypeOptions Freq: Power/Freq
      mask TypeOptions Vinit: Power/Vinit
      mask TypeOptions Iinit: Power/Iinit
      mask TypeOptions Ts: Power/Ts
  Power Factor1 : Display
  Scope : Scope
  Scope2 : Scope
  THD : powerlib_meascontrol/Measurements/THD  Freq=60  Ts=Ts_Power
      settings: SourceProductName=Simscape Electrical
  THD (% and signal) : Scope  NumInputPorts=2
  THD (%) : Display
      settings: Format=bank
  Terminator : Terminator
  Vabc pu1 : Scope
  frecuency (Hz) : Display
  to % : Gain  Gain=100  SampleTime=Ts_Power
  ángulo de V (%)1 : Display
      settings: Format=bank
  "Means_Bus8      " : Outport
  tag scope: PFabc_Bus8=global, THDv_abc_Bus8=global, delta_abc_Bus8=global
  wires:
  [IabcLL_Bus_8] -> Power Factor Block1/2(Iabc), Mux/2  "Iabc"
  THD/1 -> to %/1
  Mux/1 -> "Means_Bus8      "/1
  Power Factor Block1/4(Iabc y Iabc (rms)) -> Measurement1/4
  Power Factor Block1/1(Pabc) -> Measurement1/1
  Conv pu1/1 -> Vabc pu1/1
  Power Factor Block1/2(Qabc) -> Measurement1/2
  Power Factor Block1/3(Vabc y Vabc (rms)) -> Conv pu1/1, Measurement1/3
  to %/1 -> [THDv_abc_Bus8], THD (%)/1, THD (% and signal)/2  "THD (%)"
  Power Factor Block1/5("PFabc ") -> [PFabc_Bus8], Power Factor1/1
  PLL/1(delta_abc) -> [delta_abc_Bus8], Scope/1, ángulo de V (%)1/1
  Conv pu2/1 -> PLL/1(Vabc_LN_pu)
  PLL (3ph)/2 -> Terminator/1
  PLL (3ph)/1 -> Scope2/1, frecuency (Hz)/1
  [VabcLL_Bus_8] -> Power Factor Block1/1(Vabc), Mux/1, Conv pu2/1, PLL (3ph)/1, THD/1, THD (% and signal)/1  "Vabc"

== system Model_14Bus_Microgrid_R2018/Bus_9 ==
  note: C
  note: B
  note: A
  note: C
  note: Linea - Neutro
  note: B
  note: A
  note: A
  note: B
  Conv pu1 : Gain  Gain=sqrt (3) /Vnom_prim  SaturateOnIntegerOverflow=on  OutDataTypeStr=Inherit: Same as input  ParamDataTypeStr=Inherit: Same as input
  Conv pu2 : Gain  Gain=sqrt (3) /Vnom_prim  SaturateOnIntegerOverflow=on  OutDataTypeStr=Inherit: Same as input  ParamDataTypeStr=Inherit: Same as input
  Measurement1 : Scope  NumInputPorts=4
  PLL : Subsystem
  Power Factor Block1 : Subsystem  mask(Power Factor Block){Freq=Fnom, Vinit=[0, 0], Iinit=[0, 0], Ts=0}
      mask prompts: Freq "Fundamental frequency (Hz):"; Vinit "Voltage initial input [ Mag, Phase (degrees) ]:"; Iinit "Current initial input [ Mag, Phase (degrees) ]:"; Ts "Sample time:"
      mask help:
      | Power Factor Block developed by Dr Rodney Tan
      | Version 1.01 (Aug 2016)
      |
      | Compute power factor and phase angle of AC circuit voltage-current pair at fundamental frequency.
      |
      | The computation is based on Power block and Complex number function block.
      |
      | For the first cycle of simulation, the outputs are held constant to the powers computed for the Voltage initial input and Current initial input parameters.
      mask Help:
      | <b>Fundamental Frequency (Hz)</b>
      | Specify the measurement fundamental frequency, in hertz, of the input signal.
      | 
      | <b>Voltage initial input [ Mag, Phase (degrees) ]</b>
      | Specify the voltage initial magnitude and phase to set a constant output for the first cycle of simulation.
      | 
      | <b>Current initial input [ Mag, Phase (degrees) ]</b>
      | Specify the current initial magnitude and phase to set a constant output for the first cycle of simulation.
      | 
      | <b>Sample Time</b>
      | Specify the sample time of the block, in seconds. Set to 0 to implement a continuous block.
      mask TypeOptions Freq: Power/Freq
      mask TypeOptions Vinit: Power/Vinit
      mask TypeOptions Iinit: Power/Iinit
      mask TypeOptions Ts: Power/Ts
  Power Factor1 : Display
  Scope : Scope
  THD : powerlib_meascontrol/Measurements/THD  Freq=60  Ts=Ts_Power
      settings: SourceProductName=Simscape Electrical
  THD (% and signal) : Scope  NumInputPorts=2
  THD (%) : Display
      settings: Format=bank
  Vabc pu1 : Scope
  to % : Gain  Gain=100  SampleTime=Ts_Power
  ángulo de V (%)1 : Display
      settings: Format=bank
  tag scope: PFabc_Bus9=global, THDv_abc_Bus9=global, delta_abc_Bus9=global
  wires:
  [IabcLL_Bus_9] -> Power Factor Block1/2(Iabc)
  THD/1 -> to %/1
  Power Factor Block1/4(Iabc y Iabc (rms)) -> Measurement1/4
  Power Factor Block1/1(Pabc) -> Measurement1/1
  Conv pu1/1 -> Vabc pu1/1
  Power Factor Block1/2(Qabc) -> Measurement1/2
  Power Factor Block1/3(Vabc y Vabc (rms)) -> Conv pu1/1, Measurement1/3
  to %/1 -> [THDv_abc_Bus9], THD (%)/1, THD (% and signal)/2  "THD (%)"
  Power Factor Block1/5("PFabc ") -> [PFabc_Bus9], Power Factor1/1
  PLL/1(delta_abc) -> [delta_abc_Bus9], Scope/1, ángulo de V (%)1/1
  [VabcLL_Bus_9] -> Conv pu2/1, THD/1, THD (% and signal)/1, Power Factor Block1/1(Vabc)  "Signal Vabc"
  Conv pu2/1 -> PLL/1(Vabc_LN_pu)

== system Model_14Bus_Microgrid_R2018/Bus_AC PV  ==
  note: C
  note: B
  note: A
  note: C
  note: Linea - Neutro
  note: B
  note: A
  note: B
  note: A
  note: C
  Conv pu1 : Gain  Gain=sqrt (3) /Vnom_prim  SaturateOnIntegerOverflow=on  OutDataTypeStr=Inherit: Same as input  ParamDataTypeStr=Inherit: Same as input
  Conv pu2 : Gain  Gain=sqrt (3) /Vnom_prim  SaturateOnIntegerOverflow=on  OutDataTypeStr=Inherit: Same as input  ParamDataTypeStr=Inherit: Same as input
  Measurement1 : Scope  NumInputPorts=4
  PLL : Subsystem
  PLL (3ph) : powerlib_meascontrol/PLL/PLL (3ph)  Fmin=45  Par_Init=[0, 60]  ParK=[180, 3200, 1]  TcD=1e-4  MaxRateChangeFreq=12  FilterCutOffFreq=25  Ts=0  AGC=on
      settings: SourceProductName=Simscape Electrical
  Power Factor Block1 : Subsystem  mask(Power Factor Block){Freq=Fnom, Vinit=[0, 0], Iinit=[0, 0], Ts=0}
      mask prompts: Freq "Fundamental frequency (Hz):"; Vinit "Voltage initial input [ Mag, Phase (degrees) ]:"; Iinit "Current initial input [ Mag, Phase (degrees) ]:"; Ts "Sample time:"
      mask help:
      | Power Factor Block developed by Dr Rodney Tan
      | Version 1.01 (Aug 2016)
      |
      | Compute power factor and phase angle of AC circuit voltage-current pair at fundamental frequency.
      |
      | The computation is based on Power block and Complex number function block.
      |
      | For the first cycle of simulation, the outputs are held constant to the powers computed for the Voltage initial input and Current initial input parameters.
      mask Help:
      | <b>Fundamental Frequency (Hz)</b>
      | Specify the measurement fundamental frequency, in hertz, of the input signal.
      | 
      | <b>Voltage initial input [ Mag, Phase (degrees) ]</b>
      | Specify the voltage initial magnitude and phase to set a constant output for the first cycle of simulation.
      | 
      | <b>Current initial input [ Mag, Phase (degrees) ]</b>
      | Specify the current initial magnitude and phase to set a constant output for the first cycle of simulation.
      | 
      | <b>Sample Time</b>
      | Specify the sample time of the block, in seconds. Set to 0 to implement a continuous block.
      mask TypeOptions Freq: Power/Freq
      mask TypeOptions Vinit: Power/Vinit
      mask TypeOptions Iinit: Power/Iinit
      mask TypeOptions Ts: Power/Ts
  Power Factor1 : Display
  Scope : Scope
  Scope2 : Scope
  THD : powerlib_meascontrol/Measurements/THD  Freq=60  Ts=Ts_Power
      settings: SourceProductName=Simscape Electrical
  THD (% and signal) : Scope  NumInputPorts=2
  THD (%) : Display
      settings: Format=bank
  Terminator : Terminator
  Vabc pu1 : Scope
  frecuency (Hz) : Display
  to % : Gain  Gain=100  SampleTime=Ts_Power
  ángulo de V (%)1 : Display
      settings: Format=bank
  wires:
  [Iabc_B1] -> Power Factor Block1/2(Iabc)
  THD/1 -> to %/1
  to %/1 -> THD (%)/1, THD (% and signal)/2  "THD (%)"
  Power Factor Block1/4(Iabc y Iabc (rms)) -> Measurement1/4
  Power Factor Block1/1(Pabc) -> Measurement1/1
  Conv pu1/1 -> Vabc pu1/1
  Power Factor Block1/5("PFabc ") -> Power Factor1/1
  Power Factor Block1/2(Qabc) -> Measurement1/2
  Power Factor Block1/3(Vabc y Vabc (rms)) -> Conv pu1/1, Measurement1/3
  Conv pu2/1 -> PLL/1(Vabc_LN_pu)
  PLL/1(delta_abc) -> Scope/1, ángulo de V (%)1/1
  PLL (3ph)/1 -> Scope2/1, frecuency (Hz)/1
  PLL (3ph)/2 -> Terminator/1
  [Vabc_B1] -> Power Factor Block1/1(Vabc), PLL (3ph)/1, Conv pu2/1, THD/1, THD (% and signal)/1  "Vabc"

== system Model_14Bus_Microgrid_R2018/Bus_AC//DC3 ==
  note: BUS
  Battery system : Subsystem
      mask Display: disp('Open this block\nto display additional \nscopes & measurements')
  Conv pu1 : Gain  Gain=1 /Vnom_DC  SaturateOnIntegerOverflow=on  OutDataTypeStr=Inherit: Same as input  ParamDataTypeStr=Inherit: Same as input
  Display6 : Display
  Gain : Gain  Gain=-2/1000
  Mean : powerlib_meascontrol/Measurements/Mean  Freq=10  Vinit=0  Ts=0
      settings: SourceProductName=Simscape Electrical
  Mux : Mux  Inputs=2
  PV system : Subsystem
      mask Display: disp('Open this block\nto display additional \nscopes & measurements')
  Product : Product
  Scope3 : Scope  NumInputPorts=3
  tag scope: P_BusDC=global, V_pu_BusDC=global
  wires:
  Conv pu1/1 -> Scope3/1, [V_pu_BusDC]  "DC Voltage (pu)"
  [Vdc_bus] -> Product/1, Conv pu1/1
  [I_BusDC] -> Mux/1, Mean/1  "instant current DC (A)"
  Mean/1 -> Product/2, Mux/2, Display6/1  "Current mean DC (A)"
  Product/1 -> Gain/1
  Mux/1 -> Scope3/3
  Gain/1 -> Scope3/2, [P_BusDC]  "Power (kW)"
